simulink model "FG_Simulator"  (R2017b)
settings: Solver=VariableStepAuto  StartTime=0  StopTime=20  FixedStep=0.0005  EnableMultiTasking=on
InitFcn:
  | isSim = 1;
  | PreFunctions.CustomInitFcn;
  | PreFunctions.simulationInitFcn
values from neighbouring files (symbols this model uses):
  s = min(s_unsat,1.05)    [FG_Controller.m]
undefined symbols (not defined in the file or in its folder): DiagnosticCodes, fcut_velocity_joint, GaitLibrary, motorPositions, motorVelocities, pelvisPosition, pelvisVelocity, UserParams, X, Y, Z
libraries: slrtlib x113, sm_lib x12, nesl_utility x7, CassieLibrary x3, simulink x1, func_block_library x1
(part 1 of 3)
settings Model: Creator=case  LastModifiedBy=haoyu
settings SolverCC: ZeroCrossControl=DisableAll  InsertRTBMode=Always
settings DataIOCC: SaveOutput=off  SignalLogging=off  DSMLogging=off  SaveTime=off
settings OptimizationCC: DefaultParameterBehavior=Inlined  UseFloatMulNetSlope=on  InlineInvariantSignals=on  EfficientFloat2IntCast=on  LifeSpan=inf  SimCompilerOptimization=on  AccelVerboseBuild=on
settings DebuggingCC: ReadBeforeWriteMsg=DisableAll  WriteAfterWriteMsg=DisableAll  WriteAfterReadMsg=DisableAll  ParameterUnderflowMsg=error  ParameterTunabilityLossMsg=error  UniqueDataStoreMsg=error  AllowSymbolicDim=off  StrictBusMsg=ErrorOnBusTreatedAsVector  SFUnexpectedBacktrackingDiag=warning  SFNoUnconditionalDefaultTransitionDiag=warning  SFExecutionAtInitializationDiag=none
settings HardwareCC: TargetBitPerPointer=64  TargetBitPerSizeT=64  TargetBitPerPtrDiffT=64  TargetLongLongMode=on  TargetIntDivRoundTo=Zero  TargetEndianess=LittleEndian  TargetWordSize=64  TargetHWDeviceType=MATLAB Host  ProdEqTarget=off
settings ModelReferenceCC: EnableParallelModelReferenceBuilds=on  ModelReferenceNumInstancesAllowed=Zero  ModelReferenceMinAlgLoopOccurrences=on  PropagateSignalLabelsOutOfModel=off
settings SFSimCC: SimUserIncludeDirs=D:\Graduate\robots\Cassie\GitHub\Cassie_Controller_V3_Yukai\Controllers\Flatground\utils\funcs\kin
settings SFSimCC: SimUserSources=|
  | ComPosition_src.c
  | ComVelocity_src.c
  | J_LeftToeBottomBack_src.c
  | J_LeftToeBottomFront_src.c
  | J_LeftToeBottom_src.c
  | J_LeftToeJoint_src.c
  | J_RightToeBottomBack_src.c
  | J_RightToeBottomFront_src.c
  | J_RightToeBottom_src.c
  | J_RightToeJoint_src.c
  | LeftToeBottomBack_src.c
  | LeftToeBottomFront_src.c
  | LeftToeBottom_src.c
  | LeftToeJoint_src.c
  | RightToeBottomBack_src.c
  | RightToeBottomFront_src.c
  | RightToeBottom_src.c
  | RightToeJoint_src.c
settings RTWCC: Description=Generic Real-Time Target  RTWUseSimCustomCode=on  CustomInclude=D:\Graduate\robots\Cassie\GitHub\Cassie_Controller_V3_Yukai\Controllers\Flatground\utils\funcs\kin  BuildConfiguration=Faster Runs  CheckMdlBeforeBuild=Warning
settings RTWCC: CustomSource=|
  | ComPosition_src.c
  | ComVelocity_src.c
  | J_LeftToeBottomBack_src.c
  | J_LeftToeBottomFront_src.c
  | J_LeftToeBottom_src.c
  | J_LeftToeJoint_src.c
  | J_RightToeBottomBack_src.c
  | J_RightToeBottomFront_src.c
  | J_RightToeBottom_src.c
  | J_RightToeJoint_src.c
  | LeftToeBottomBack_src.c
  | LeftToeBottomFront_src.c
  | LeftToeBottom_src.c
  | LeftToeJoint_src.c
  | RightToeBottomBack_src.c
  | RightToeBottomFront_src.c
  | RightToeBottom_src.c
  | RightToeJoint_src.c
settings CodeAppCC: GenerateComments=off  SimulinkBlockComments=off
settings GRTTargetCC: MatFileLogging=off  MultiInstanceERTCode=on  CodeInterfacePackaging=Reusable function  SupportNonFinite=off  GenerateAllocFcn=on
settings ConfigComp: CovMetricSettings=dw  CovHtmlReporting=on  CovSaveCumulativeToWorkspaceVar=on  CovSaveSingleToWorkspaceVar=on  CovExternalEMLEnable=off
settings SimscapeCC: SimscapeNormalizeSystem=off
settings DiagnosticsConfigSet: SimMechanicsRigidlyBoundBlock=warning
settings ExplorerConfigSet: InternalSimMechanicsExplorerSettings="<ExplorerConfiguration><canonicalview>default</canonicalview><AnimationSetting><BasePlaybackSpeed>1.0</BasePlaybackSpeed><PlaybackSpeedFactor>1.0</PlaybackSpeedFactor></AnimationSetting><TilePanel><TileInfo><Tiles Columns=\"1\" Count=\"1\" Rows=\"1\"><Column Weight=\"1\"/><Row Weight=\"1\"/><Tile Height=\"1\" Width=\"1\" X=\"0\" Y=\"0\"/></Tiles></TileInfo><SceneInfo><SceneViewer><BGColor><R>0.60000002384185791</R><G>0.60000002384185791</G><B>0.60000002384185791</B></BGColor><Camera><DoPerspective>on</DoPerspective><Position><X>1.49424103443841916</X><Y>-1.5003618867302666</Y><Z>-0.448846928440659099</Z></Position><Center><X>-0.00575896556158084216</X><Y>-0.000361886730266602896</Y><Z>-0.948846928440659099</Z></Center><Up><X>0</X><Y>0</Y><Z>1</Z></Up><ViewLimDist>1</ViewLimDist><YLim>0.466307658154998583</YLim><XLim>2.07568807125632082</XLim></Camera></SceneViewer></SceneInfo></TilePanel><MechEditorPanel><Cameras><Camera><Id>Camera1</Id><Value><Name>Tracking Camera</Name><NativeCamera><PositionTrackingFeature>Cassie.Cassie_Simulation.World.Tracking_Camera.F</PositionTrackingFeature><CenterTrackingFeature>Cassie.Cassie_Simulation.World.Tracking_Camera_Target.F</CenterTrackingFeature><UpVectorTrackingFeature>Cassie.Cassie_Simulation.World.Tracking_Camera_Target.F</UpVectorTrackingFeature><CenterTrackingOrigin>on</CenterTrackingOrigin><UpVectorTrackingDirection>+Z</UpVectorTrackingDirection></NativeCamera></Value></Camera><Camera><Id>Camera2</Id><Value><Name>Fixed Camera</Name><NativeCamera><PositionTrackingFeature>Cassie.Cassie_Simulation.World.Fixed_Camera.F</PositionTrackingFeature><CenterTrackingFeature>Cassie.Cassie_Simulation.World.Fixed_Camera_Target.F</CenterTrackingFeature><UpVectorTrackingFeature>Cassie.Cassie_Simulation.World.Fixed_Camera_Target.F</UpVectorTrackingFeature><CenterTrackingOrigin>on</CenterTrackingOrigin><UpVectorTrackingDirection>+Z</UpVectorTrackingDirection></NativeCamera></Value></Camera></Cameras><GfxPanelCameraMap><MapElement CameraMLId=\"Camera1\" GfxPanelIndex=\"0\"/></GfxPanelCameraMap><VideoCreator><PlaybackSpeedRatio>1.0</PlaybackSpeedRatio><FrameRate>30</FrameRate><VideoFormat>Motion JPEG AVI</VideoFormat><FrameSize>auto</FrameSize></VideoCreator></MechEditorPanel></ExplorerConfiguration>"

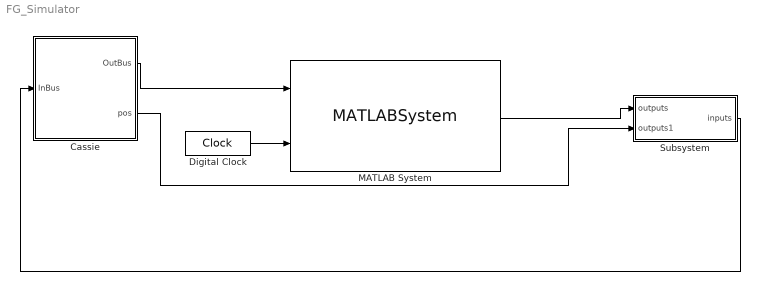
== system FG_Simulator ==
  Cassie : Subsystem  AncestorBlock=CassieLibrary/Simulation/Cassie  InitFcn=|  StartFcn=|  StopFcn=|
      InitFcn=|
      | % Start clock at initialization (used for computing real time performance)
      | initTime = tic;
      | 
      | % Import bus definitions
      | CassieModule.importBuses;
      StartFcn=|
      | % Store build time
      | buildTime = toc(initTime);
      StopFcn=|
      | % Store computation time
      | computationTime = toc(initTime) - buildTime;
      | 
      | % Get simulation time
      | simulationTime = get_param(bdroot, 'SimulationTime');
      | 
      | % Compute real time performance
      | percentRealTime = 100*simulationTime/computationTime;
      | 
      | % Display
      | fprintf('Build time: %0.2f seconds \n', buildTime);
      | fprintf('Simulation time: %0.2f seconds \n', simulationTime);
      | fprintf('Computation time: %0.2f seconds \n', computationTime);
      | fprintf('Performance: %0.2f%% real time \n', percentRealTime);
      mask Display: image('Cassie.png');
  Digital Clock : DigitalClock  SampleTime=UserParams.SampleTime
  MATLAB System : MATLABSystem  System=RemoteSpoofer  SimulateUsing=Code generation
      mask Type: RemoteSpoofer
      mask Display:
      | disp('RemoteSpoofer');
      | port_label('input',1,'cassieOutputs');
      | port_label('input',2,'t');
      | port_label('output',1,'cassieOutputs');
  Subsystem : Subsystem  AncestorBlock=FG_Controller_Library/Subsystem
  wires:
  Cassie/1(OutBus) -> MATLAB System/1
  Digital Clock/1 -> MATLAB System/2
  MATLAB System/1 -> Subsystem/1(outputs)
  Subsystem/1("inputs ") -> Cassie/1(InBus)
  Cassie/2(pos) -> Subsystem/2(outputs1)

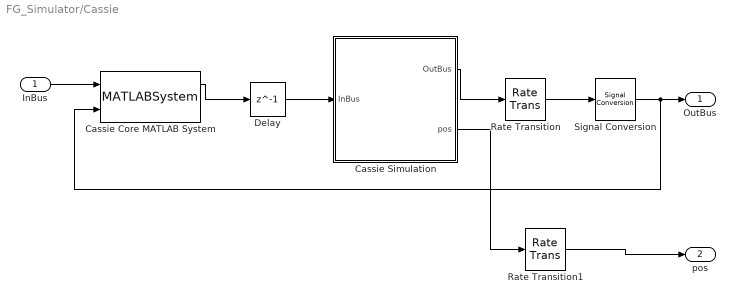
== system FG_Simulator/Cassie ==
  InBus : Inport  OutDataTypeStr=Bus: CassieUserInBus
  Cassie Core MATLAB System : MATLABSystem  System=CassieCoreSim  SimulateUsing=Code generation
      mask Type: CassieCoreSim
      mask Display: disp('CassieCoreSim');
  Cassie Simulation : Subsystem  AncestorBlock=CassieLibrary/Simulation/Cassie Simulation
      mask Display: image('Cassie.png');
  Delay : Delay  DelayLength=1
  Rate Transition : RateTransition  OutPortSampleTime=0.0005
  Rate Transition1 : RateTransition  OutPortSampleTime=0.0005
  Signal Conversion : SignalConversion  ConversionOutput=Nonvirtual bus  OutDataTypeStr=Bus: CassieOutBus  OverrideOpt=off
  OutBus : Outport  OutDataTypeStr=Bus: CassieOutBus
  pos : Outport  Port=2
  wires:
  Signal Conversion/1 -> OutBus/1, Cassie Core MATLAB System/2
  Cassie Simulation/1(OutBus) -> Rate Transition/1
  Rate Transition/1 -> Signal Conversion/1
  Delay/1 -> Cassie Simulation/1(InBus)
  Cassie Core MATLAB System/1 -> Delay/1
  InBus/1 -> Cassie Core MATLAB System/1
  Rate Transition1/1 -> pos/1
  Cassie Simulation/2(pos) -> Rate Transition1/1

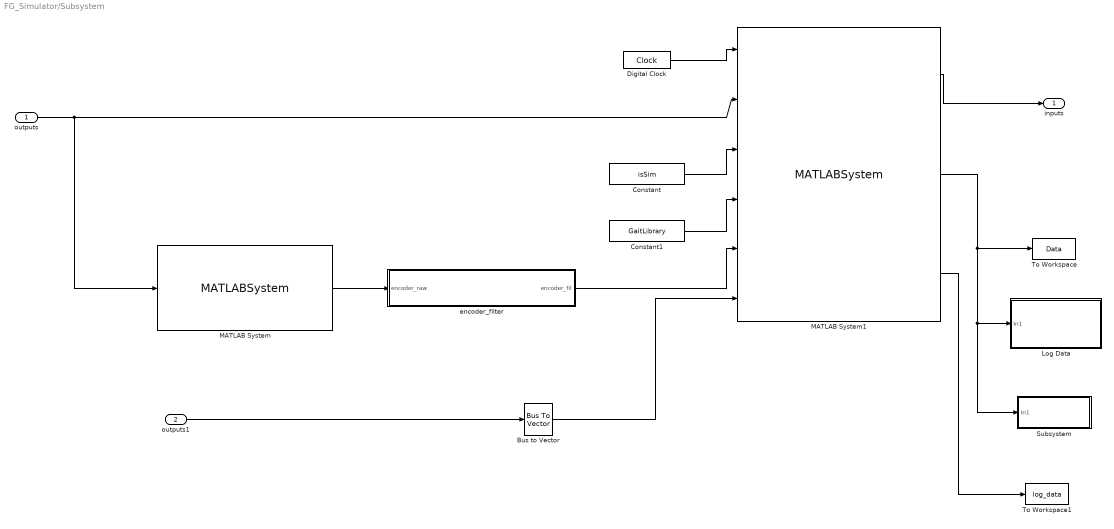
== system FG_Simulator/Subsystem ==
  outputs : Inport  OutDataTypeStr=Bus: CassieOutBus
  outputs1 : Inport  Port=2
  Bus to Vector : BusToVector
  Constant : Constant  Value=isSim  OutDataTypeStr=boolean  LockScale=on
  Constant1 : Constant  Value=GaitLibrary  OutDataTypeStr=Bus: cassieGaitLibraryBus  LockScale=on
  Digital Clock : DigitalClock  SampleTime=UserParams.SampleTime
  Log Data : Subsystem
  MATLAB System : MATLABSystem  System=ExtractJointPosition  SimulateUsing=Code generation
      mask Type: ExtractJointPosition
      mask Display:
      | disp('ExtractJointPosition');
      | port_label('input',1,'cassieOutputs');
      | port_label('output',1,'JointPosition');
  MATLAB System1 : MATLABSystem  System=FG_Controller  Kp_pitch=c_Kp_pitch  Kd_pitch=c_Kd_pitch  Kp_roll=c_Kp_roll  Kd_roll=c_Kd_roll  Kp_yaw=c_Kp_yaw  Kd_yaw=c_Kd_yaw  Kp_abduction=c_Kp_abduction  Kp_rotation=c_Kp_rotation  Kp_thigh=c_Kp_thigh  Kp_knee=c_Kp_knee  Kp_toe=c_Kp_toe  Kd_abduction=c_Kd_abduction  Kd_rotation=c_Kd_rotation  Kd_thigh=c_Kd_thigh  Kd_knee=c_Kd_knee  Kd_toe=c_Kd_toe  Kfs_p=c_Kfs_p  Kfl_p=c_Kfl_p  Kfs_d=c_Kfs_d  Kfl_d=c_Kfl_d  Kp_toe_stand=c_Kp_toe_stand  Kd_toe_stand=c_Kd_toe_stand  Kp_lateral_stand=c_Kp_lateral_stand  Kd_lateral_stand=c_Kd_lateral_stand  Kp_abduction_stand=c_Kp_abduction_stand  Kd_abduction_stand=c_Kd_abduction_stand  Kp_thigh_stand=c_Kp_thigh_stand  Kd_thigh_stand=c_Kd_thigh_stand  Kp_knee_stand=c_Kp_knee_stand  Kd_knee_stand=c_Kd_knee_stand  Kp_rotation_stand=c_Kp_rotation_stand  Kd_rotation_stand=c_Kd_rotation_stand  fil_para_x=c_fil_para_x  fil_para_y=c_fil_para_y  stance_thre_ub=c_stance_thre_ub  stance_thre_lb=c_stance_thre_lb  lateral_velocity_weight=c_lateral_velocity_weight  init_lateral_velocity=c_init_lateral_velocity  abduction_inward_gain=c_abduction_inward_gain  joint_filter_choice=c_joint_filter_choice  shift_time=c_shift_time  shift_distance=c_shift_distance  standing_switch_time=c_standing_switch_time  toe_tilt_angle=c_toe_tilt_angle  final_sw_abduction=c_final_sw_abduction  final_st_abduction=c_final_st_abduction  pre_final_sw_abduction=c_pre_final_sw_abduction  sagittal_offset_exp=c_sagittal_offset_exp  lateral_offset_exp=c_lateral_offset_exp  turning_offset_exp=c_turning_offset_exp  stand_offset_exp=c_stand_offset_exp  u_abduction_cp=c_u_abduction_cp  u_abduction_swing_cp=c_u_abduction_swing_cp  u_thigh_cp=c_u_thigh_cp  u_knee_cp=c_u_knee_cp  fil_para_2=c_fil_para_2  fil_para_3=c_fil_para_3  fil_para_4=c_fil_para_4  fil_para_5=c_fil_para_5  force_step_end_s=c_force_step_end_s  SimulateUsing=Code generation
      mask Type: FG_Controller
      mask Display:
      | disp('FG_Controller');
      | port_label('input',1,'t');
      | port_label('input',2,'cassieOutputs');
      | port_label('input',3,'isSim');
      | port_label('input',4,'GaitLibrary');
      | port_label('input',5,'encoder_fil');
      | port_label('input',6,'pos');
      | port_label('output',1,'userInputs');
      | port_label('output',2,'Data');
      | port_label('output',3,'log_data');
  Subsystem : Subsystem
  To Workspace : ToWorkspace  VariableName=Data  SaveFormat=Timeseries  SampleTime=-1
  To Workspace1 : ToWorkspace  VariableName=log_data  SaveFormat=Timeseries  SampleTime=-1
  encoder_filter : Subsystem  TreatAsAtomicUnit=on
  "inputs " : Outport
  wires:
  Constant1/1 -> MATLAB System1/4
  Constant/1 -> MATLAB System1/3
  Digital Clock/1 -> MATLAB System1/1
  MATLAB System1/2 -> To Workspace/1, Log Data/1(In1), Subsystem/1(In1)
  MATLAB System1/1 -> "inputs "/1
  encoder_filter/1(encoder_fil) -> MATLAB System1/5
  MATLAB System/1 -> encoder_filter/1(encoder_raw)
  outputs/1 -> MATLAB System/1, MATLAB System1/2
  outputs1/1 -> Bus to Vector/1
  Bus to Vector/1 -> MATLAB System1/6
  MATLAB System1/3 -> To Workspace1/1

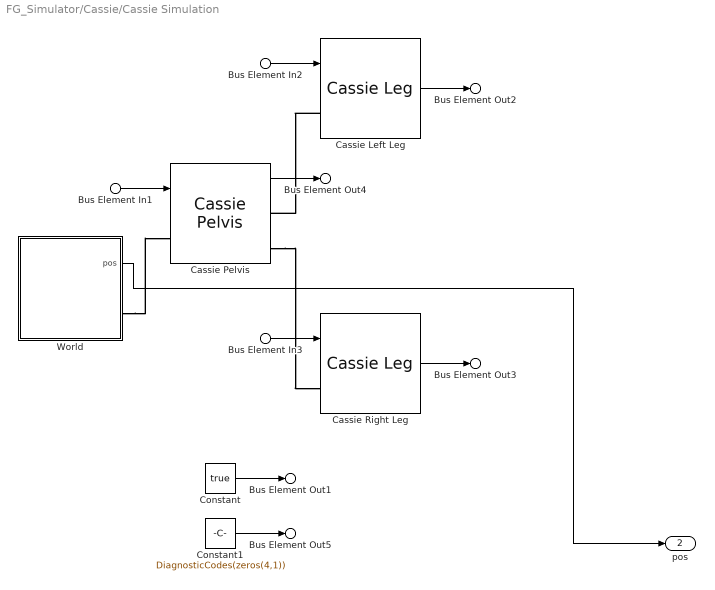
== system FG_Simulator/Cassie/Cassie Simulation ==
  Bus Element In2 : Inport  PortName=InBus  Element=leftLeg
  Bus Element In3 : Inport  PortName=InBus  Element=rightLeg
  Bus Element In1 : Inport  PortName=InBus  Element=pelvis
  Cassie Left Leg : CassieLibrary/Simulation/Cassie Leg  config=Left  motorPositions=motorPositions(1:5)  motorVelocities=motorVelocities(1:5)
  Cassie Pelvis : CassieLibrary/Simulation/Cassie Pelvis  SystemSampleTime=-1
  Cassie Right Leg : CassieLibrary/Simulation/Cassie Leg  config=Right  motorPositions=motorPositions(6:10)  motorVelocities=motorVelocities(6:10)
  Constant : Constant  Value=true
  Constant1 : Constant  Value=DiagnosticCodes(zeros(4,1))
  World : Subsystem  AncestorBlock=ComponentLibrary/Simulation/World
  Bus Element Out4 : Outport  PortName=OutBus  Element=pelvis
  Bus Element Out2 : Outport  PortName=OutBus  Element=leftLeg
  Bus Element Out3 : Outport  PortName=OutBus  Element=rightLeg
  Bus Element Out1 : Outport  PortName=OutBus  Element=isCalibrated
  Bus Element Out5 : Outport  PortName=OutBus  Element=messages
  pos : Outport  Port=2
  wires:
  Constant1/1 -> Bus Element Out5/1
  Constant/1 -> Bus Element Out1/1
  Bus Element In1/1 -> Cassie Pelvis/1
  Cassie Right Leg/1 -> Bus Element Out3/1
  Bus Element In2/1 -> Cassie Left Leg/1
  Cassie Left Leg/1 -> Bus Element Out2/1
  Bus Element In3/1 -> Cassie Right Leg/1
  Cassie Pelvis/1 -> Bus Element Out4/1
  World/1(pos) -> pos/1
  connections:
  World/RConn1 -- Cassie Pelvis/LConn1
  Cassie Left Leg/LConn1 -- Cassie Pelvis/RConn1
  Cassie Pelvis/RConn2 -- Cassie Right Leg/LConn1

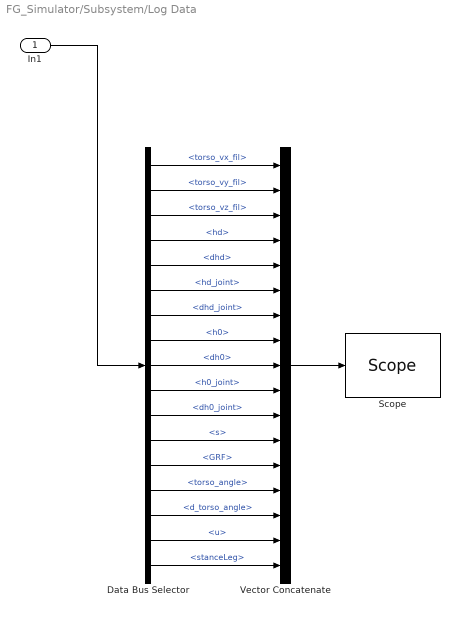
== system FG_Simulator/Subsystem/Log Data ==
  In1 : Inport  OutDataTypeStr=Bus: cassieDataBus
  Data Bus Selector : BusSelector  OutputSignals=torso_vx_fil,torso_vy_fil,torso_vz_fil,hd,dhd,hd_joint,dhd_joint,h0,dh0,h0_joint,dh0_joint,s,GRF,torso_angle,d_torso_angle,u,stanceLeg
  "Scope " : slrtlib/Displays and Logging/Scope   scopeno=5  scopetype=File  autostart=on  viewmode=Graphical redraw  formatstr='%15.6f'  grid=on  ylimits=[0,0]  nosamples=250  noprepostsamples=0  interleave=1  triggermode=FreeRun  triggersignal=1  trigsignalfromport=off  triggerlevel=0.0  triggerslope=Either  triggerscope=1  triggersample=0  filename=data.dat  mode=Lazy  writesize=512*8  autorestart=on  dynamicfilemode=off  maxwritefilesize=4*1024^3
  Vector Concatenate : Concatenate  NumInputs=17
  wires:
  Data Bus Selector/17 -> Vector Concatenate/17  "<stanceLeg>"
  Data Bus Selector/16 -> Vector Concatenate/16  "<u>"
  Data Bus Selector/12 -> Vector Concatenate/12  "<s>"
  Data Bus Selector/11 -> Vector Concatenate/11  "<dh0_joint>"
  Data Bus Selector/15 -> Vector Concatenate/15  "<d_torso_angle>"
  Data Bus Selector/14 -> Vector Concatenate/14  "<torso_angle>"
  Data Bus Selector/13 -> Vector Concatenate/13  "<GRF>"
  Data Bus Selector/4 -> Vector Concatenate/4  "<hd>"
  Data Bus Selector/5 -> Vector Concatenate/5  "<dhd>"
  Data Bus Selector/1 -> Vector Concatenate/1  "<torso_vx_fil>"
  Data Bus Selector/6 -> Vector Concatenate/6  "<hd_joint>"
  Data Bus Selector/2 -> Vector Concatenate/2  "<torso_vy_fil>"
  Data Bus Selector/3 -> Vector Concatenate/3  "<torso_vz_fil>"
  Data Bus Selector/10 -> Vector Concatenate/10  "<h0_joint>"
  Data Bus Selector/9 -> Vector Concatenate/9  "<dh0>"
  Data Bus Selector/8 -> Vector Concatenate/8  "<h0>"
  Data Bus Selector/7 -> Vector Concatenate/7  "<dhd_joint>"
  Vector Concatenate/1 -> "Scope "/1
  In1/1 -> Data Bus Selector/1
